simulink model "tableXOpenloopPositionModel"  (R2016b)
settings: Solver=ode15s  StartTime=0.0  StopTime=2.0015  RelTol=1e-3
settings Model: Creator=chenb  LastModifiedBy=chenb

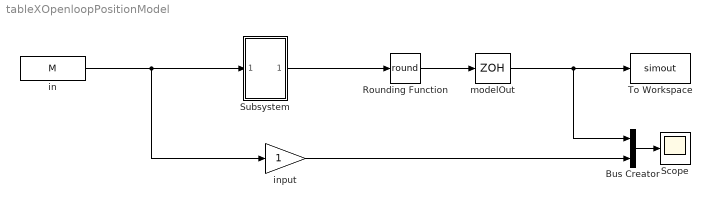
== system tableXOpenloopPositionModel ==
  Bus Creator : BusCreator  Inputs=2
  Rounding Function : Rounding  Operator=round
  Scope : Scope
  Subsystem : Subsystem
  To Workspace : ToWorkspace  VariableName=simout  SampleTime=0.00025
  in : FromWorkspace  VariableName=M  SampleTime=0.00025
  input : Gain
  modelOut : ZeroOrderHold  SampleTime=0.00025
  wires:
  input/1 -> Bus Creator/2
  Subsystem/1(Out1) -> Rounding Function/1
  Bus Creator/1 -> Scope/1
  Rounding Function/1 -> modelOut/1
  modelOut/1 -> To Workspace/1, Bus Creator/1
  in/1 -> input/1, Subsystem/1(In1)

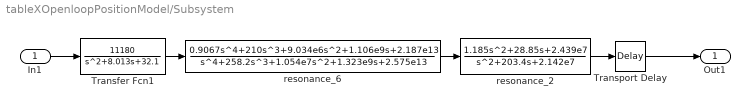
== system tableXOpenloopPositionModel/Subsystem ==
  In1 : Inport
  Transfer Fcn1 : TransferFcn  Numerator=[11180]  Denominator=[1 8.013 32.1]
  Transport Delay : TransportDelay  DelayTime=0.001
  resonance_2 : TransferFcn  Numerator=[1.185 28.85 2.439e7]  Denominator=[1 203.4 2.142e7]
  resonance_6 : TransferFcn  Numerator=[0.9067 210 9.034e6 1.106e9 2.187e13]  Denominator=[1 258.2 1.054e7 1.323e9 2.575e13]
  Out1 : Outport
  wires:
  Transfer Fcn1/1 -> resonance_6/1
  resonance_2/1 -> Transport Delay/1
  resonance_6/1 -> resonance_2/1
  In1/1 -> Transfer Fcn1/1
  Transport Delay/1 -> Out1/1
